simulink model "perrottaC1"  (R2020b)
settings: Solver=FixedStepDiscrete  StartTime=0.0  StopTime=200  FixedStep=Ts  RelTol=1e-3
model workspace (MAT data in the model file):
  Ts = 0.002
  acoeff = 0.95
  amax = 0.1
  jcoeff = 0.1
  jmax = 1
  pf = 160
  reference_command = [0 0.002 0.004 0.006 0.008 0.01 0.012 0.014 0.016 0.018 0.02 0.022 ... (200002 elements, 100001x2)]
  v = 50
  vmax = 1.5
libraries: simulink x3
(part 1 of 2)
settings Model: Creator=rspp  LastModifiedBy=savar
settings DataIOCC: ExternalInput=az,alt,rot

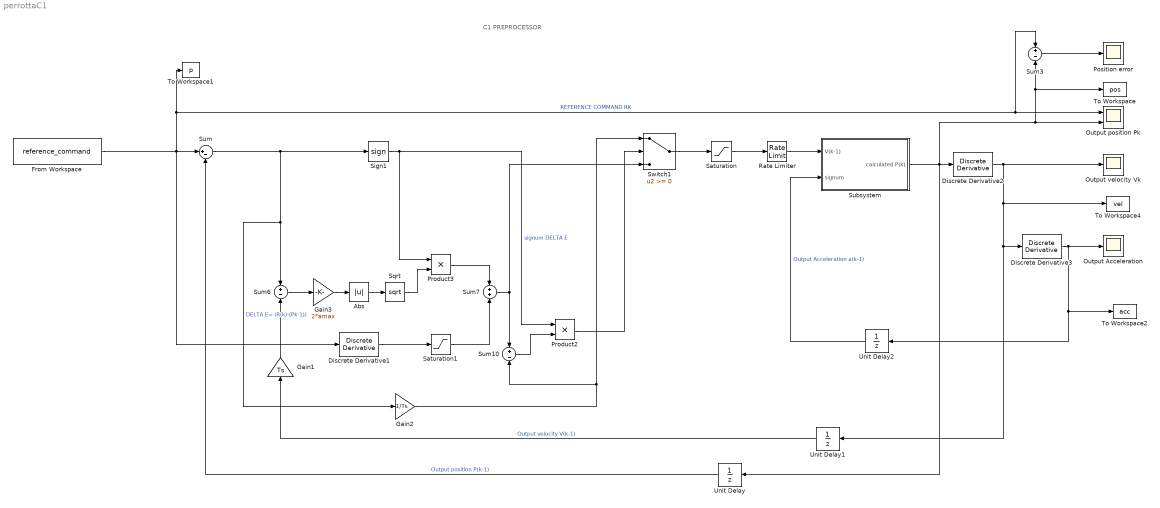
== system perrottaC1 ==
  note: C1 PREPROCESSOR
  Abs : Abs
  Discrete Derivative1 : simulink/Discrete/Discrete Derivative  gainval=1.0  ICPrevScaledInput=0.0  OutMin=[]  OutMax=[]  OutDataType=fixdt(1, 16)  OutScaling=2^-10  DoSatur=off
  Discrete Derivative2 : simulink/Discrete/Discrete Derivative  gainval=1.0  ICPrevScaledInput=0.0  OutMin=[]  OutMax=[]  OutDataType=fixdt(1, 16)  OutScaling=2^-10  DoSatur=off
  Discrete Derivative3 : simulink/Discrete/Discrete Derivative  gainval=1.0  ICPrevScaledInput=0.0  OutMin=[]  OutMax=[]  OutDataType=fixdt(1, 16)  OutScaling=2^-10  DoSatur=off
  From Workspace : FromWorkspace  VariableName=reference_command
  Gain1 : Gain  Gain=Ts
  Gain2 : Gain  Gain=1/Ts
  Gain3 : Gain  Gain=2*amax
  Output Acceleration : Scope
  Output position Pk : Scope  NumInputPorts=2
  Output velocity Vk : Scope
  Position error : Scope
  Product2 : Product
  Product3 : Product
  Rate Limiter : RateLimiter  RisingSlewLimit=amax  FallingSlewLimit=-amax  SampleTimeMode=inherited
  Saturation : Saturate  UpperLimit=vmax  LowerLimit=-vmax
  Saturation1 : Saturate  UpperLimit=vmax  LowerLimit=-vmax
  Sign1 : Signum
  Sqrt : Sqrt  SaturateOnIntegerOverflow=on
  Subsystem : Subsystem
  Sum : Sum  Inputs=|+-
  Sum10 : Sum  Inputs=+-
  Sum3 : Sum  Inputs=+-
  Sum6 : Sum  Inputs=+-
  Sum7 : Sum
  Switch1 : Switch
  To Workspace : ToWorkspace  VariableName=pos  SampleTime=-1
  To Workspace1 : ToWorkspace  VariableName=p  SampleTime=-1
  To Workspace2 : ToWorkspace  VariableName=acc  SampleTime=-1
  To Workspace4 : ToWorkspace  VariableName=vel  SampleTime=-1
  Unit Delay : UnitDelay  SampleTime=-1  HasFrameUpgradeWarning=on
  Unit Delay1 : UnitDelay  SampleTime=-1  HasFrameUpgradeWarning=on
  Unit Delay2 : UnitDelay  SampleTime=-1  HasFrameUpgradeWarning=on
  wires:
  Sum/1 -> Gain2/1, Sum6/1, Sign1/1  "DELTA E= (R(k)-(Pk-1))"
  From Workspace/1 -> Sum/1, To Workspace1/1, Sum3/1, Output position Pk/1, Discrete Derivative1/1  "REFERENCE COMMAND RK"
  Subsystem/1(calculated P(k)) -> Unit Delay/1, Discrete Derivative2/1, To Workspace/1, Sum3/2, Output position Pk/2
  Saturation/1 -> Rate Limiter/1
  Unit Delay/1 -> Sum/2  "Output position P(k-1)"
  Abs/1 -> Sqrt/1
  Discrete Derivative2/1 -> To Workspace4/1, Unit Delay1/1, Discrete Derivative3/1, Output velocity Vk/1
  Gain3/1 -> Abs/1
  Switch1/1 -> Saturation/1
  Unit Delay1/1 -> Gain1/1  "Output velocity V(k-1)"
  Gain2/1 -> Switch1/1, Sum10/2
  Discrete Derivative1/1 -> Saturation1/1
  Gain1/1 -> Sum6/2
  Sign1/1 -> Product3/1, Product2/1  "signum DELTA E"
  Sum7/1 -> Switch1/3, Sum10/1
  Sqrt/1 -> Product3/2
  Product3/1 -> Sum7/1
  Sum10/1 -> Product2/2
  Sum3/1 -> Position error/1
  Saturation1/1 -> Sum7/2
  Sum6/1 -> Gain3/1
  Product2/1 -> Switch1/2
  Rate Limiter/1 -> Subsystem/1(V(k-1))
  Discrete Derivative3/1 -> Output Acceleration/1, Unit Delay2/1, To Workspace2/1
  Unit Delay2/1 -> Subsystem/2(signum)  "Output Acceleration a(k-1)"
